simulink model "dspanc1"  (R2023b)
settings: Solver=FixedStepDiscrete  StartTime=0.0  StopTime=inf  RelTol=1e-3  EnableMultiTasking=on
libraries: dspvision x1, audiosources x1, dspsrcs4 x1, dspsnks4 x1, dspadpt3 x1
settings Model: Creator=The MathWorks, Inc.  LastModifiedBy=jawad
settings SolverCC: AlgebraicLoopSolver=TrustRegion  MaxZcPerStep=1
settings DataIOCC: SaveFormat=Array  SaveOutput=off  SaveTime=off  ReturnWorkspaceOutputs=off  SignalLoggingName=sigsOut
settings OptimizationCC: ExpressionDepthLimit=2147483647  InitFltsAndDblsToZero=on  EfficientMapNaN2IntZero=off  LifeSpan=inf  SimCompilerOptimization=on
settings DebuggingCC: UnderspecifiedInitializationDetection=Classic  MergeDetectMultiDrivingBlocksExec=none  CheckExecutionContextPreStartOutputMsg=on  SignalResolutionControl=TryResolveAllWithWarning  MultiTaskDSMMsg=warning  MultiTaskCondExecSysMsg=none  ParameterPrecisionLossMsg=none  FcnCallInpInsideContextMsg=warning  UnconnectedInputMsg=warning  UnconnectedOutputMsg=warning  UnconnectedLineMsg=warning  AllowSymbolicDim=off  StateNameClashWarn=warning  SymbolicDimsDataTypeCodeGenerationDiagnostic=none  SFUnexpectedBacktrackingDiag=warning  SFNoUnconditionalDefaultTransitionDiag=warning  SFExecutionAtInitializationDiag=none  ArithmeticOperatorsInVariantConditions=warning
settings HardwareCC: ProdBitPerPointer=32  ProdBitPerSizeT=32  ProdBitPerPtrDiffT=32  ProdLargestAtomicFloat=None  ProdIntDivRoundTo=Undefined  ProdEndianess=Unspecified  ProdWordSize=32  ProdHWDeviceType=32-bit Generic  TargetUnknown=on
settings ModelReferenceCC: UpdateModelReferenceTargets=IfOutOfDate  EnableRefExpFcnMdlSchedulingChecks=on  PropagateSignalLabelsOutOfModel=off
settings SFSimCC: SimUseLocalCustomCode=off  CustomCodeUndefinedFunction=UseInterfaceOnly
settings RTWCC: RTWUseLocalCustomCode=off  DLArmComputeVersion=19.05
settings CodeAppCC: StateflowObjectComments=on
settings GRTTargetCC: TargetFcnLib=ansi_tfl_tmw_new.mat  TargetLangStandard=C89/C90 (ANSI)  CombineOutputUpdateFcns=off  GRTInterface=on
settings ConfigComp: CovMetricSettings=dw  CovSaveCumulativeToWorkspaceVar=on  CovSaveSingleToWorkspaceVar=on  CovExternalEMLEnable=off  CovSFcnEnable=off

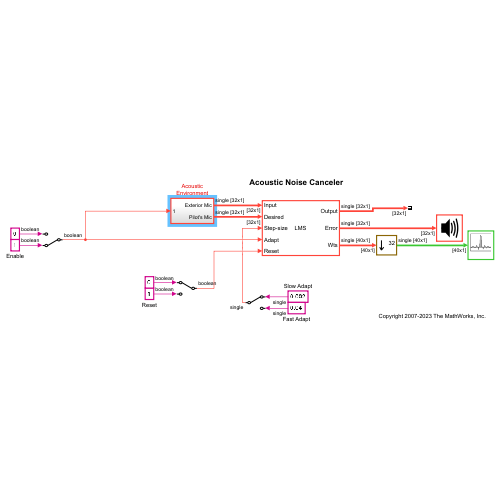
[thumbnail: Simulink's stored preview of the top-level diagram]
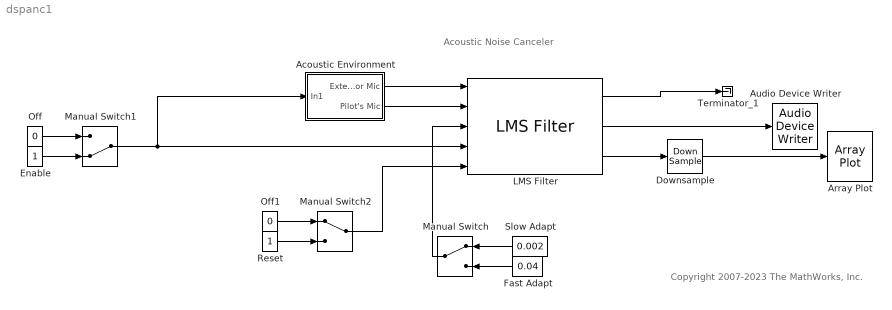
== system dspanc1 ==
  note: Acoustic Noise Canceler
  note: Copyright 2007-2023 The MathWorks, Inc.
  Acoustic Environment : Subsystem
  Array Plot : ArrayPlot  WindowPosition=[770.000000,50.000000,766.000000,785.000000,]  Visible=on  ScopeFrameLocation=window  XLabel=Samples  YLimits=[-0.0744 0.2746]
  Audio Device Writer : dspsnks4/Audio Device Writer  Driver=DirectSound  Device=Speakers (Realtek(R) Audio)  InheritSampleRate=on  SampleRate=44100  BitDepth=16-bit integer  BufferSize=4096  NumBuffers=10  DefaultOutputChannelMapping=on  OutputChannelMapping=1:2  OutputNumUnderrunSamples=off  DriverIdx=1  DeviceWarnFlag=''
  Downsample : DownSample  N=32  RateOptions=Allow multirate processing
  Enable : Constant  OutDataTypeStr=boolean
  Fast Adapt : Constant  Value=0.04  OutDataTypeStr=Inherit: Inherit via back propagation
  LMS Filter : dspadpt3/LMS Filter  Algo=LMS  L=40  stepflag=Input port  mu=0.1  leakage=1.0  ic=0  Adapt=on  resetflag=Non-zero sample  weights=on  addnparflag=off  roundingMode=Floor  overflowMode=off  secondCoeffMode=Binary point scaling  secondCoeffWordLength=2  secondCoeffFracLength=15  prodOutput2Mode=Binary point scaling  prodOutput2FracLength=20  prodOutput3Mode=Binary point scaling  prodOutput3FracLength=20  prodOutput4Mode=Binary point scaling  prodOutput4FracLength=20  quotientMode=Binary point scaling  quotientFracLength=20  accum2Mode=Binary point scaling  accum2FracLength=20
  Manual Switch : ManualSwitch
  Manual Switch1 : ManualSwitch  CurrentSetting=0
  Manual Switch2 : ManualSwitch
  Off : Constant  Value=0  OutDataTypeStr=boolean
  Off1 : Constant  Value=0  OutDataTypeStr=boolean
  Reset : Constant  OutDataTypeStr=boolean
  Slow Adapt : Constant  Value=0.002  OutDataTypeStr=Inherit: Inherit via back propagation
  Terminator_1 : Terminator
  wires:
  Downsample/1 -> Array Plot/1
  Acoustic Environment/1(Exterior Mic) -> LMS Filter/1
  Slow Adapt/1 -> Manual Switch/1
  Fast Adapt/1 -> Manual Switch/2
  Manual Switch/1 -> LMS Filter/3
  LMS Filter/3 -> Downsample/1
  Acoustic Environment/2(Pilot's Mic) -> LMS Filter/2
  LMS Filter/2 -> Audio Device Writer/1
  LMS Filter/1 -> Terminator_1/1
  Off/1 -> Manual Switch1/1
  Enable/1 -> Manual Switch1/2
  Off1/1 -> Manual Switch2/1
  Reset/1 -> Manual Switch2/2
  Manual Switch2/1 -> LMS Filter/5
  Manual Switch1/1 -> Acoustic Environment/1(In1), LMS Filter/4

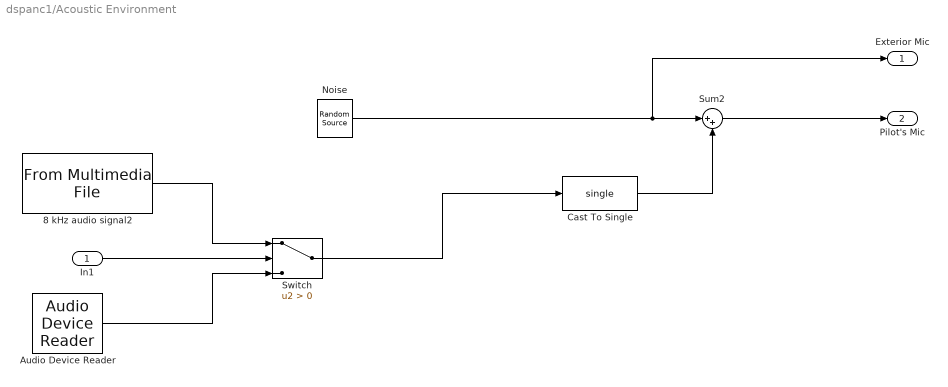
== system dspanc1/Acoustic Environment ==
  In1 : Inport
  8 kHz audio signal2 : dspvision/From Multimedia File  inputFilename=C:\Users\jawad\MATLAB\Senior Design\AcousticNoiseCancellationLMSExample\noisy.wav  readRange=[1 Inf]  loop=on  numPlays=inf  outputStreams=Audio only  videoDataType=single  audioDataType=single  inheritSampleTime=on  userDefinedSampleTime=1/30  noAudioOutput=off  isIntensityVideo=off  fourcc=RGB  colorVideoFormat=Separate color signals  outputEOF=off  dataOrg=Column-major  audioFrameSize=32  computeAudioFrameSize=off  outSamplingMode=Sample based
  Audio Device Reader : audiosources/Audio Device Reader  Driver=DirectSound  Device=Default  SampleRate=22050  NumChannels=1  SamplesPerFrame=32  BitDepth=16-bit integer  NumBuffers=10  DefaultInputChannelMapping=on  InputChannelMapping=1:2  OutputNumOverrunSamples=off  OutputDataType=single  DriverIdx=1  DeviceWarnFlag=''
  Cast To Single : DataTypeConversion  OutDataTypeStr=single  SaturateOnIntegerOverflow=off  RndMeth=Floor
  Noise : dspsrcs4/Random Source  SrcType=Gaussian  NormMethod=Sum of uniform values  CltLength=5  MinVal=-1  MaxVal=1  MeanVal=0  VarVal=1  RepMode=Specify seed  rawSeed=[23341]  IsInherit=off  SampMode=Discrete  SampTime=1/22050  SampFrame=32  DataType=Single  OutComplex=Real  OutputFrames=off
  Sum2 : Sum  Inputs=|++  InputSameDT=on  SaturateOnIntegerOverflow=on  OutDataTypeStr=Inherit: Same as first input
  Switch : Switch  Criteria=u2 > Threshold  SaturateOnIntegerOverflow=off  InputSameDT=off
  Exterior Mic : Outport  VectorParamsAs1DForOutWhenUnconnected=off
  Pilot's Mic : Outport  Port=2  VectorParamsAs1DForOutWhenUnconnected=off
  wires:
  Cast To Single/1 -> Sum2/2
  Sum2/1 -> Pilot's Mic/1
  Noise/1 -> Exterior Mic/1, Sum2/1
  In1/1 -> Switch/2
  Switch/1 -> Cast To Single/1
  Audio Device Reader/1 -> Switch/3
  8 kHz audio signal2/1 -> Switch/1
